simulink model "ASM_Traffic_V2X_Complete_Model_2"  (R2019a)
settings: Solver=ode1  StartTime=SIM.tstart.v  StopTime=Inf  FixedStep=SIM.StepSize.v  RelTol=1e-3
PostLoadFcn:
  | if any(exist('dsrtsu_mdlpostloadfcn', 'file') ~= 0), dsrtsu_mdlpostloadfcn('Execute', bdroot); end
  | try, asm_mdl_postloadfcn(bdroot, 'UpdateModel', 2200); catch, disp(lasterr); end,
undefined symbols (not defined in the file): _SensorPnts_1, _SensorPnts_13, _SensorPnts_17, _SensorPnts_21, _SensorPnts_25, _SensorPnts_29, _SensorPnts_33, _SensorPnts_37, _SensorPnts_41, _SensorPnts_45, _SensorPnts_49, _SensorPnts_5, _SensorPnts_53, _SensorPnts_57, _SensorPnts_9, _to_, CPT, G5A, ITS, MDL, rad, s_to_rpm, SIM
libraries: simulink x169, ASM_VehicleDynamics_lib x126, ASM_Traffic_lib x83, ASM_Utils_lib x49, mdbs x45, ASM_Environment_lib x17, dspindex x12, dsaV2xLibraryAux x10, dsmpblib x6, dsaV2xAsn1Library x4, dsaV2xLibrary x4, ASM_BrakeHydraulics_lib x4
(part 20 of 36)

== system ASM_Traffic_V2X_Complete_Model_2/MDL/Environment/Traffic/Sensors/Custom_Sensor ==
  Fellows_Signals : Inport
  VehicleDynamics_Signals : Inport  Port=2
  Objects_Signals : Inport  Port=3
  Road_Signals : Inport  Port=4
  ASMSignalBus_Mapping : Subsystem
  ASMSignalCollector : Subsystem
  Bus Creator4 : BusCreator  Inputs=1
  Bus Selector : BusSelector  OutputSignals=TrafficObject_Type_Fellows[],TrafficObject_Type_Data[]
  Bus Selector2 : BusSelector  OutputSignals=TrafficObject_Data[]
  Bus Selector3 : BusSelector  OutputSignals=VehicleMovement.Positions.Pos_Vehicle_CoorSys_E[x;y;z][m].Pos_Vehicle_CoorSys_E[x;y;z][m],VehicleMovement.Positions.Angle_Vehicle_CoorSys_E[x;y;z][deg].Angle_Vehicle_CoorSys_E[x;y;z][deg]
  Bus Selector4 : BusSelector  OutputSignals=Pos_Fellows_MainPnt_CoorSys_E[x;y;z][m],Angle_Fellows[x;y;z][deg],Flag_FellowUsed[0|1]
  CUSTOM_SENSOR_GEOMETRY_PARAMETERS : ASM_Traffic_lib/Sensors/Custom_Sensor/CUSTOM_SENSOR_GEOMETRY_PARAMETERS  Tag=ASM_SUBCOMPONENT  Sensor_Enable=MDL.Traffic.Sensors.CustomSensor_Geometry.Sw_Sensor_Enable  Pos_Sensor=MDL.Traffic.Sensors.CustomSensor_Geometry.Const_Pos_Sensor_Apex_CoorSys_V  Angle_Orientation_Sensor=MDL.Traffic.Sensors.CustomSensor_Geometry.Const_Angle_Orientation_Sensor_CoorSys_V  Length_ScopeZone=MDL.Traffic.Sensors.CustomSensor_Geometry.Const_Length_ScopeZone  Angle_ScopeZone_Horizontal=MDL.Traffic.Sensors.CustomSensor_Geometry.Const_Angle_ScopeZone_Horizontal  Angle_ScopeZone_Vertical=MDL.Traffic.Sensors.CustomSensor_Geometry.Const_Angle_ScopeZone_Vertical  ASMProperties=struct('Name','CUSTOM_SENSOR_GEOMETRY_PARAMETERS','Version','2.0','Library','ASM_Traffic_lib')  ASMInstanceName=custom_sensor_geometry_parameters  ASMInstanceID=1
  CUSTOM_SENSOR_OUTPUT : ASM_Traffic_lib/Sensors/Custom_Sensor/CUSTOM_SENSOR_OUTPUT  Tag=ASM_SUBCOMPONENT  ASMProperties=struct('Name','CUSTOM_SENSOR_OUTPUT','Version','4.0','Library','ASM_Traffic_lib')  ASMInstanceName=custom_sensor_output  ASMInstanceID=1
  CUSTOM_SENSOR_SCOPEZONE_CALCULATION : ASM_Traffic_lib/Sensors/Custom_Sensor/CUSTOM_SENSOR_SCOPEZONE_CALCULATION  Tag=ASM_SUBCOMPONENT  ASMProperties=struct('Name','CUSTOM_SENSOR_SCOPEZONE_CALCULATION','Version','4.0','Library','ASM_Traffic_lib')  ASMInstanceName=custom_sensor_scopezone_calculation  ASMInstanceID=1
  Enable_Custom_Sensor : Subsystem
  SensorOutput_Mapping : Subsystem
  TrafficObject_Type : Subsystem
  Vector Concatenate : Concatenate  NumInputs=5
  Sensor_Signals : Outport
  tag scope: ASMBUS_Environment_Traffic_Sensors_Custom_Sensor_1=global, ASMBUS_Environment_Traffic_Sensors_Custom_Sensor_1_Parameters=global
  wires:
  Enable_Custom_Sensor/1(Enable_Out[0Off|1On]) -> CUSTOM_SENSOR_SCOPEZONE_CALCULATION/1
  CUSTOM_SENSOR_GEOMETRY_PARAMETERS/1 -> [ASMBUS_Environment_Traffic_Sensors_Custom_Sensor_1_Parameters]
  TrafficObject_Type/1(Out1) -> CUSTOM_SENSOR_OUTPUT/1
  ASMSignalBus_Mapping/1(ASMSignalBus) -> [ASMBUS_Environment_Traffic_Sensors_Custom_Sensor_1]
  Bus Creator4/1 -> Sensor_Signals/1
  SensorOutput_Mapping/1(Sensor_Signals) -> Bus Creator4/1  "Sensor_Front_1"
  CUSTOM_SENSOR_OUTPUT/2 -> SensorOutput_Mapping/2(ObjectData)
  CUSTOM_SENSOR_SCOPEZONE_CALCULATION/1 -> ASMSignalBus_Mapping/1(ScopezoneData)
  Bus Selector4/1 -> CUSTOM_SENSOR_SCOPEZONE_CALCULATION/5  "<Pos_Fellows_MainPnt_CoorSys_E[x;y;z][m]>"
  CUSTOM_SENSOR_GEOMETRY_PARAMETERS/2 -> Enable_Custom_Sensor/1(Enable_In[0Off|1On])
  CUSTOM_SENSOR_GEOMETRY_PARAMETERS/7 -> Vector Concatenate/5
  CUSTOM_SENSOR_GEOMETRY_PARAMETERS/6 -> Vector Concatenate/4
  CUSTOM_SENSOR_GEOMETRY_PARAMETERS/5 -> Vector Concatenate/3
  CUSTOM_SENSOR_GEOMETRY_PARAMETERS/4 -> Vector Concatenate/2
  CUSTOM_SENSOR_GEOMETRY_PARAMETERS/3 -> Vector Concatenate/1
  Bus Selector4/3 -> CUSTOM_SENSOR_SCOPEZONE_CALCULATION/7  "<Flag_FellowUsed[0|1]>"
  Bus Selector4/2 -> CUSTOM_SENSOR_SCOPEZONE_CALCULATION/6  "<Angle_Fellows[x;y;z][deg]>"
  Bus Selector3/2 -> CUSTOM_SENSOR_SCOPEZONE_CALCULATION/4  "<Angle_Vehicle_CoorSys_E[x;y;z][deg]>"
  Bus Selector3/1 -> CUSTOM_SENSOR_SCOPEZONE_CALCULATION/3  "<Pos_Vehicle_CoorSys_E[x;y;z][m]>"
  Bus Selector2/1 -> CUSTOM_SENSOR_SCOPEZONE_CALCULATION/10  "<TrafficObject_Data[]>"
  Vector Concatenate/1 -> CUSTOM_SENSOR_SCOPEZONE_CALCULATION/2
  Bus Selector/1 -> CUSTOM_SENSOR_SCOPEZONE_CALCULATION/8  "<TrafficObject_Type_Fellows[]>"
  CUSTOM_SENSOR_SCOPEZONE_CALCULATION/2 -> TrafficObject_Type/1(In1), SensorOutput_Mapping/1(ScopezoneData)
  CUSTOM_SENSOR_OUTPUT/1 -> ASMSignalBus_Mapping/2(ObjectData)
  Bus Selector/2 -> CUSTOM_SENSOR_OUTPUT/2, CUSTOM_SENSOR_SCOPEZONE_CALCULATION/9  "<TrafficObject_Type_Data[]>"
  Fellows_Signals/1 -> Bus Selector4/1
  VehicleDynamics_Signals/1 -> Bus Selector3/1
  Objects_Signals/1 -> Bus Selector/1
  Road_Signals/1 -> Bus Selector2/1

== system ASM_Traffic_V2X_Complete_Model_2/MDL/Environment/Traffic/Sensors/Line_Sensor ==
  Enable[0Off|1On] : Inport
  VehicleDynamics_Signals : Inport  Port=2
  Road_Signals : Inport  Port=3
  Maneuver_Signals : Inport  Port=4
  ASMSignalCollector : Subsystem
  Bus Selector1 : BusSelector  OutputSignals=VehicleMovement.Positions.Pos_Vehicle_CoorSys_E[x;y;z][m].Pos_x_Vehicle_CoorSys_E[m],VehicleMovement.Positions.Pos_Vehicle_CoorSys_E[x;y;z][m].Pos_y_Vehicle_CoorSys_E[m],VehicleMovement.Positions.Angle_Vehicle_CoorSys_E[x;y;z][deg].Angle_Yaw_Vehicle_CoorSys_E[deg]
  Bus Selector5 : BusSelector  OutputSignals=MdlControl.Reset_VehicleStates[0|1],Info.ManeuverState[],InitialVehStates.Route_Id_Init[],InitialVehStates.Route_Direction_Init[]
  Bus Selector6 : BusSelector  OutputSignals=Road_ASMVeh.s_Veh_Road[m],Road_Info.d_Veh_Ref_Line[m]
  Enable_Line_Sensor : Subsystem
  LINE_SENSOR : ASM_Traffic_lib/Sensors/Line_Sensor/LINE_SENSOR  Tag=ASM_SUBCOMPONENT  Const_Length_Sensor_Range=MDL.Traffic.Sensors.LineSensor.Const_Length_Sensor_Range  Const_Num_Lines_Per_Side_Max=MDL.Traffic.Sensors.LineSensor.Const_Num_Lines_Per_Side_Max  Const_Dist_Road_Sample_Pnts=MDL.Traffic.Sensors.LineSensor.Const_Dist_Road_Sample_Pnts  Const_Road_Lane_Output_Dimension=MDL.Traffic.Sensors.LineSensor.Const_Road_Lane_Output_Dimension  Const_Road_Shape_Line_Output_Dimension=MDL.Traffic.Sensors.LineSensor.Const_Road_Shape_Line_Output_Dimension  Const_Road_Shape_ContObj_Output_Dimension=MDL.Traffic.Sensors.LineSensor.Const_Road_Shape_ContObj_Output_Dimension  Const_Junction_Border_Output_Dimension=MDL.Traffic.Sensors.LineSensor.Const_Junction_Border_Output_Dimension  Const_Junction_Shape_Line_Output_Dimension=MDL.Traffic.Sensors.LineSensor.Const_Junction_Shape_Line_Output_Dimension  Const_Junction_Shape_ContObj_Output_Dimension=MDL.Traffic.Sensors.LineSensor.Const_Junction_Shape_ContObj_Output_Dimension  Sw_Sensor_Enable=MDL.Traffic.Sensors.LineSensor.Sw_Sensor_Enable  ASMProperties=struct('Name','LINE_SENSOR','Version','5.0','Library','ASM_Traffic_lib')  ASMInstanceName=line_sensor  ASMInstanceID=1
  Sensor_Signals : Outport
  tag scope: ASMBUS_Traf_Sensors_Line_Sensor_1=global
  wires:
  Enable_Line_Sensor/1(Enable_Out[0Off|1On]) -> LINE_SENSOR/1
  Bus Selector6/2 -> LINE_SENSOR/8  "<d_Veh_Ref_Line[m]>"
  Bus Selector1/3 -> LINE_SENSOR/11  "<Angle_Yaw_Vehicle_CoorSys_E[deg]>"
  Bus Selector1/2 -> LINE_SENSOR/10  "<Pos_y_Vehicle_CoorSys_E[m]>"
  Bus Selector1/1 -> LINE_SENSOR/9  "<Pos_x_Vehicle_CoorSys_E[m]>"
  VehicleDynamics_Signals/1 -> Bus Selector1/1
  Bus Selector6/1 -> LINE_SENSOR/7  "<s_Veh_Road[m]>"
  Road_Signals/1 -> Bus Selector6/1
  Bus Selector5/4 -> LINE_SENSOR/6  "<Route_Direction_Init[]>"
  Bus Selector5/3 -> LINE_SENSOR/5  "<Route_Id_Init[]>"
  Bus Selector5/2 -> LINE_SENSOR/4  "<ManeuverState[]>"
  Bus Selector5/1 -> LINE_SENSOR/3  "<Reset_VehicleStates[0|1]>"
  Maneuver_Signals/1 -> Bus Selector5/1
  Enable[0Off|1On]/1 -> Enable_Line_Sensor/1(Enable_In[0Off|1On])
  [ASM_Environment_LineSensorData] -> LINE_SENSOR/2
  LINE_SENSOR/2 -> Sensor_Signals/1
  LINE_SENSOR/1 -> [ASMBUS_Traf_Sensors_Line_Sensor_1]

== system ASM_Traffic_V2X_Complete_Model_2/MDL/Environment/Traffic/Sensors/Object_Sensor_2D ==
  Enable[0Off|1On] : Inport
  Fellows_Signals : Inport  Port=2
  VehicleDynamics_Signals : Inport  Port=3
  Objects_Signals : Inport  Port=4
  Road_Signals : Inport  Port=5
  ASMSignalCollector : Subsystem
  Enable_Object_Sensor_2D : Subsystem
  ScheduleAndCalculateSensor : Subsystem
  SensorMapping : Subsystem
  SensorParameters : Subsystem
  Sensor_Signals : Outport
  wires:
  Enable[0Off|1On]/1 -> Enable_Object_Sensor_2D/1(Enable_In[0Off|1On])
  Enable_Object_Sensor_2D/1(Enable_Out[0Off|1On]) -> ScheduleAndCalculateSensor/2(Enable[0Off|1On]), SensorMapping/1(Enable[0Off|1On])
  SensorMapping/1(Sensor_Signals) -> Sensor_Signals/1
  VehicleDynamics_Signals/1 -> ScheduleAndCalculateSensor/4(VehicleDynamics_Signals)
  SensorParameters/1(Sensor_Data[]) -> ScheduleAndCalculateSensor/1(Sensor_Data[])
  Fellows_Signals/1 -> ScheduleAndCalculateSensor/3(Fellows_Signals)
  Objects_Signals/1 -> ScheduleAndCalculateSensor/5(Objects_Signals)
  Road_Signals/1 -> ScheduleAndCalculateSensor/6(Road_Signals)
  ScheduleAndCalculateSensor/1(SensorMapping_Data[]) -> SensorMapping/2(SensorMapping_Data[])
  ScheduleAndCalculateSensor/2(SensorSignals) -> SensorMapping/3(SensorSignals)

== system ASM_Traffic_V2X_Complete_Model_2/MDL/Environment/Traffic/Sensors/Object_Sensor_3D ==
  Enable[0Off|1On] : Inport
  Fellows_Signals : Inport  Port=2
  VehicleDynamics_Signals : Inport  Port=3
  Objects_Signals : Inport  Port=4
  Road_Signals : Inport  Port=5
  ASMSignalCollector : Subsystem
  CustomPoints : Subsystem
  Enable_Object_Sensor_3D : Subsystem
  RadarEffects : Subsystem
  ScheduleAndCalculateSensor : Subsystem
  SensorMapping : Subsystem
  SensorParameters : Subsystem
  Sensor_Signals : Outport
  wires:
  ScheduleAndCalculateSensor/5(Pos_Vehicle_CoorSys_E_Sampled[x,y;z][m]) -> RadarEffects/5(Pos_Vehicle_CoorSys_E[x;y;z][m])
  ScheduleAndCalculateSensor/4(Angle_Vehicle_CoorSys_E_Sampled[x,y;z][deg]) -> RadarEffects/4(Angle_Vehicle_CoorSys_E[x;y;z][deg])
  ScheduleAndCalculateSensor/3(SensorData[]) -> RadarEffects/3(SensorData[]), CustomPoints/3(SensorData[])
  Enable[0Off|1On]/1 -> Enable_Object_Sensor_3D/1(Enable_In[0Off|1On])
  Enable_Object_Sensor_3D/1(Enable_Out[0Off|1On]) -> ScheduleAndCalculateSensor/2(Enable[0Off|1On]), SensorMapping/1(Enable[0Off|1On]), RadarEffects/1(Enable[0Off|1On]), CustomPoints/1(Enable[0Off|1On])
  SensorMapping/1(Sensor_Signals) -> Sensor_Signals/1
  VehicleDynamics_Signals/1 -> ScheduleAndCalculateSensor/4(VehicleDynamics_Signals)
  SensorParameters/1(Sensor_Data[]) -> ScheduleAndCalculateSensor/1(Sensor_Data[])
  Fellows_Signals/1 -> ScheduleAndCalculateSensor/3(Fellows_Signals)
  Objects_Signals/1 -> ScheduleAndCalculateSensor/5(Objects_Signals)
  Road_Signals/1 -> ScheduleAndCalculateSensor/6(Road_Signals)
  ScheduleAndCalculateSensor/1(SensorMapping_Data[]) -> SensorMapping/2(SensorMapping_Data[]), RadarEffects/2(SensorMapping_Data[]), CustomPoints/2(SensorMapping_Data[])
  ScheduleAndCalculateSensor/2(SensorSignals) -> SensorMapping/3(SensorSignals)

== system ASM_Traffic_V2X_Complete_Model_2/MDL/Environment/Traffic/Sensors/Sensors_Common_Signals ==
  Maneuver_Signals[] : Inport
  Brake : RelationalOperator  Operator===  OutDataTypeStr=boolean  RndMeth=Nearest
  Bus Selector7 : BusSelector  OutputSignals=Info.ManeuverState[]  OutputAsBus=on
  Constant : Constant  Value=3
  Constant1 : Constant  Value=4
  Data Type Conversion : DataTypeConversion  OutDataTypeStr=double
  Delay : Subsystem
  Logical Operator : Logic  Operator=OR  AllPortsSameDT=off  OutDataTypeStr=boolean
  Run : RelationalOperator  Operator===  OutDataTypeStr=boolean  RndMeth=Nearest
  SignalCollector : Subsystem
  ASMSignalBus : Outport
  Enable_Sensor_Scheduling[0Off|1On] : Outport  Port=2
  wires:
  Data Type Conversion/1 -> Delay/1(Enable_Sensor_Scheduling_In[0Off|1On])
  Delay/1(Enable_Sensor_Scheduling_Out[0Off|1On]) -> SignalCollector/1(Enable_SensorScheduling[0Off|1On]), Enable_Sensor_Scheduling[0Off|1On]/1
  SignalCollector/1(ASMSignalBus) -> ASMSignalBus/1
  Logical Operator/1 -> Data Type Conversion/1
  Brake/1 -> Logical Operator/2
  Bus Selector7/1 -> Brake/1, Run/1
  Constant1/1 -> Brake/2
  Run/1 -> Logical Operator/1
  Constant/1 -> Run/2
  Maneuver_Signals[]/1 -> Bus Selector7/1

== system ASM_Traffic_V2X_Complete_Model_2/MDL/Environment/Traffic/Sensors/Traffic_Sign_Sensor ==
  VehicleDynamics_Signals : Inport
  Objects_Signals : Inport  Port=2
  Road_Signals : Inport  Port=3
  ASMSignalCollector : Subsystem
  Bus Selector1 : BusSelector  OutputSignals=VehicleMovement.Positions.Pos_Vehicle_CoorSys_E[x;y;z][m].Pos_Vehicle_CoorSys_E[x;y;z][m],VehicleMovement.Positions.Angle_Vehicle_CoorSys_E[x;y;z][deg].Angle_Vehicle_CoorSys_E[x;y;z][deg]
  Bus Selector2 : BusSelector  OutputSignals=TrafficObject_Type_Data[]
  Bus Selector3 : BusSelector  OutputSignals=TrafficObject_Data[]
  Enable_Traffic_Sign_Sensor : Subsystem
  Mux : Mux  Inputs=6
  Objects_DataStreams : Subsystem
  TRAFFIC_SIGN_SENSOR_DYNAMIC_CALCULATION : ASM_Traffic_lib/Sensors/Traffic_Sign_Sensor/TRAFFIC_SIGN_SENSOR_DYNAMIC_CALCULATION  Tag=ASM_SUBCOMPONENT  Const_Sensor_Output_Dimension=MDL.Traffic.Sensors.TrafficSignSensorDyn_Calculation.Const_Sensor_Output_Dimension  ASMProperties=struct('Name','TRAFFIC_SIGN_SENSOR_DYNAMIC_CALCULATION','Version','1.0','Library','ASM_Traffic_lib')  ASMInstanceName=traffic_sign_sensor_dynamic_calculation  ASMInstanceID=1
  TRAFFIC_SIGN_SENSOR_GEOMETRY_PARAMETERS : ASM_Traffic_lib/Sensors/Traffic_Sign_Sensor/TRAFFIC_SIGN_SENSOR_GEOMETRY_PARAMETERS  Tag=ASM_SUBCOMPONENT  Sensor_Enable=MDL.Traffic.Sensors.TrafficSignSensor_Geometry.Sw_Sensor_Enable  Pos_Sensor=MDL.Traffic.Sensors.TrafficSignSensor_Geometry.Const_Pos_Sensor_Apex_CoorSys_V  Angle_Orientation_Sensor=MDL.Traffic.Sensors.TrafficSignSensor_Geometry.Const_Angle_Orientation_Sensor_CoorSys_V  Length_ScopeZone=MDL.Traffic.Sensors.TrafficSignSensor_Geometry.Const_Length_ScopeZone  Angle_ScopeZone_Horizontal=MDL.Traffic.Sensors.TrafficSignSensor_Geometry.Const_Angle_ScopeZone_Horizontal  Angle_ScopeZone_Vertical=MDL.Traffic.Sensors.TrafficSignSensor_Geometry.Const_Angle_ScopeZone_Vertical  Angle_Sign_Orientation_Max=MDL.Traffic.Sensors.TrafficSignSensor_Geometry.Const_Angle_Sign_Orientation_Max  ASMProperties=struct('Name','TRAFFIC_SIGN_SENSOR_GEOMETRY_PARAMETERS','Version','2.0','Library','ASM_Traffic_lib')  ASMInstanceName=traffic_sign_sensor_geometry_parameters  ASMInstanceID=1
  Sensor_Signals : Outport
  tag scope: ASMBUS_Traf_Sensors_Traffic_Sign_Sensor_dyn_1_Parameters=global, ASMBUS_Traf_Sensors_dyn_Traffic_Sign_Sensor_1=global
  wires:
  Objects_DataStreams/1(TrafficObjects_States[]) -> TRAFFIC_SIGN_SENSOR_DYNAMIC_CALCULATION/7
  Bus Selector3/1 -> TRAFFIC_SIGN_SENSOR_DYNAMIC_CALCULATION/6  "<TrafficObject_Data[]>"
  Bus Selector2/1 -> TRAFFIC_SIGN_SENSOR_DYNAMIC_CALCULATION/5  "<TrafficObject_Type_Data[]>"
  Bus Selector1/2 -> TRAFFIC_SIGN_SENSOR_DYNAMIC_CALCULATION/4  "<Angle_Vehicle_CoorSys_E[x;y;z][deg]>"
  Bus Selector1/1 -> TRAFFIC_SIGN_SENSOR_DYNAMIC_CALCULATION/3  "<Pos_Vehicle_CoorSys_E[x;y;z][m]>"
  TRAFFIC_SIGN_SENSOR_DYNAMIC_CALCULATION/2 -> Sensor_Signals/1
  TRAFFIC_SIGN_SENSOR_DYNAMIC_CALCULATION/1 -> [ASMBUS_Traf_Sensors_dyn_Traffic_Sign_Sensor_1]
  Enable_Traffic_Sign_Sensor/1(Enable_Out[0Off|1On]) -> TRAFFIC_SIGN_SENSOR_DYNAMIC_CALCULATION/1
  TRAFFIC_SIGN_SENSOR_GEOMETRY_PARAMETERS/1 -> [ASMBUS_Traf_Sensors_Traffic_Sign_Sensor_dyn_1_Parameters]
  TRAFFIC_SIGN_SENSOR_GEOMETRY_PARAMETERS/2 -> Enable_Traffic_Sign_Sensor/1(Enable_In[0Off|1On])
  Mux/1 -> TRAFFIC_SIGN_SENSOR_DYNAMIC_CALCULATION/2
  TRAFFIC_SIGN_SENSOR_GEOMETRY_PARAMETERS/8 -> Mux/6
  TRAFFIC_SIGN_SENSOR_GEOMETRY_PARAMETERS/7 -> Mux/5
  TRAFFIC_SIGN_SENSOR_GEOMETRY_PARAMETERS/6 -> Mux/4
  TRAFFIC_SIGN_SENSOR_GEOMETRY_PARAMETERS/5 -> Mux/3
  TRAFFIC_SIGN_SENSOR_GEOMETRY_PARAMETERS/4 -> Mux/2
  TRAFFIC_SIGN_SENSOR_GEOMETRY_PARAMETERS/3 -> Mux/1
  Road_Signals/1 -> Bus Selector3/1
  Objects_Signals/1 -> Bus Selector2/1
  VehicleDynamics_Signals/1 -> Bus Selector1/1

== system ASM_Traffic_V2X_Complete_Model_2/MDL/SoftECU/Map_Inputs/Maneuver/S_R_FlipFlop ==
  S : Inport
  R : Inport  Port=2
  Demux : Demux  Outputs=2
  Logic : CombinatorialLogic  TruthTable=[0 1;1 0;0 1;0 1;1 0;1 0;0 0;0 0]
  Memory : Memory  InitialCondition=initial_condition  InheritSampleTime=on
  Mux : Mux  Inputs=3
  Q : Outport  InitialOutput=0
  !Q : Outport  Port=2  InitialOutput=1
  wires:
  Demux/2 -> !Q/1
  Demux/1 -> Memory/1, Q/1
  S/1 -> Mux/1
  R/1 -> Mux/2
  Memory/1 -> Mux/3
  Mux/1 -> Logic/1
  Logic/1 -> Demux/1

== system ASM_Traffic_V2X_Complete_Model_2/MDL/SoftECU/Map_Inputs/Maneuver/pos_edge_detection ==
  In1 : Inport
  Memory : Memory
  Relational Operator : RelationalOperator  Operator=>  OutDataTypeStr=boolean  RndMeth=Nearest
  Out1 : Outport
  wires:
  Memory/1 -> Relational Operator/2
  Relational Operator/1 -> Out1/1
  In1/1 -> Memory/1, Relational Operator/1

== system ASM_Traffic_V2X_Complete_Model_2/MDL/SoftECU/Map_Inputs/Maneuver/pos_edge_detection1 ==
  In1 : Inport
  Memory : Memory
  Relational Operator : RelationalOperator  Operator=>  OutDataTypeStr=boolean  RndMeth=Nearest
  Out1 : Outport
  wires:
  In1/1 -> Relational Operator/1, Memory/1
  Relational Operator/1 -> Out1/1
  Memory/1 -> Relational Operator/2

== system ASM_Traffic_V2X_Complete_Model_2/MDL/SoftECU/Map_Inputs/Maneuver/pos_edge_detection2 ==
  In1 : Inport
  Memory : Memory
  Relational Operator : RelationalOperator  Operator=>  OutDataTypeStr=boolean  RndMeth=Nearest
  Out1 : Outport
  wires:
  Memory/1 -> Relational Operator/2
  Relational Operator/1 -> Out1/1
  In1/1 -> Memory/1, Relational Operator/1

== system ASM_Traffic_V2X_Complete_Model_2/MDL/SoftECU/Map_Inputs/Maneuver/pos_edge_detection3 ==
  In1 : Inport
  Memory : Memory
  Relational Operator : RelationalOperator  Operator=>  OutDataTypeStr=boolean  RndMeth=Nearest
  Out1 : Outport
  wires:
  In1/1 -> Relational Operator/1, Memory/1
  Relational Operator/1 -> Out1/1
  Memory/1 -> Relational Operator/2

== system ASM_Traffic_V2X_Complete_Model_2/MDL/SoftECU/Soft_ECU_ACC/Map_Inputs/Maneuver ==
  note: Initial value is set
      | to AEBOff (3)
  ECU_Commands[] : Inport
  Reset[0|1] : Inport  Port=2
  ACC_BrakeMode_Default : Constant  Value=3
  Add : Sum  Inputs=+++
  Fcn1 : Fcn  Expr=u(1)==1020
  Fcn10 : Fcn  Expr=u(1)==1031
  Fcn2 : Fcn  Expr=u(1)==1030
  Fcn3 : Fcn  Expr=u(1)==1022
  Fcn4 : Fcn  Expr=u(1)==1021
  Fcn5 : Fcn  Expr=u(1)==1013
  Fcn6 : Fcn  Expr=u(1)==1011
  Fcn7 : Fcn  Expr=u(1)==1010
  Fcn8 : Fcn  Expr=u(1)==1012
  Fcn9 : Fcn  Expr=u(1)==1032
  Gain : Gain
  Gain1 : Gain  Gain=2
  Gain2 : Gain  Gain=3
  Logical Operator : Logic  Operator=OR  Inputs=4  AllPortsSameDT=off  OutDataTypeStr=boolean
  Memory : Memory  InitialCondition=3
  Switch : Switch  Threshold=0.5
  Switch1 : Switch  Threshold=0.5
  pos_edge_detection : Subsystem
  pos_edge_detection1 : Subsystem
  pos_edge_detection2 : Subsystem
  pos_edge_detection3 : Subsystem
  Sw_ACC_On[0Off|1On] : Outport
  Sw_ACC_Off[0Off|1On] : Outport  Port=2
  Sw_ACC_Cancel[0Off|1On] : Outport  Port=3
  Sw_ACC_Resume[0Off|1On] : Outport  Port=4
  Sw_ACC_Speed_Set[0Off|1On] : Outport  Port=5
  Sw_ACC_Speed_Increase[0Off|1On] : Outport  Port=6
  Sw_ACC_Speed_Decrease[0Off|1On] : Outport  Port=7
  Sw_ACC_BrakeMode[1Comfort|2AEBOnly|3AEBOff] : Outport  Port=8
  wires:
  Fcn6/1 -> Sw_ACC_Off[0Off|1On]/1
  Fcn7/1 -> Sw_ACC_On[0Off|1On]/1
  Fcn3/1 -> Sw_ACC_Speed_Decrease[0Off|1On]/1
  Fcn4/1 -> Sw_ACC_Speed_Increase[0Off|1On]/1
  Fcn5/1 -> Sw_ACC_Resume[0Off|1On]/1
  Fcn8/1 -> Sw_ACC_Cancel[0Off|1On]/1
  Fcn1/1 -> Sw_ACC_Speed_Set[0Off|1On]/1
  ECU_Commands[]/1 -> Fcn7/1, Fcn6/1, Fcn8/1, Fcn5/1, Fcn1/1, Fcn4/1, Fcn9/1, Fcn10/1, Fcn2/1, Fcn3/1
  Fcn9/1 -> pos_edge_detection/1(In1), Gain2/1
  Fcn10/1 -> pos_edge_detection1/1(In1), Gain1/1
  Fcn2/1 -> pos_edge_detection2/1(In1), Gain/1
  pos_edge_detection/1(Out1) -> Logical Operator/1
  pos_edge_detection1/1(Out1) -> Logical Operator/2
  pos_edge_detection2/1(Out1) -> Logical Operator/3
  Gain2/1 -> Add/3
  Gain1/1 -> Add/2
  Gain/1 -> Add/1
  Logical Operator/1 -> Switch/2
  Switch/1 -> Sw_ACC_BrakeMode[1Comfort|2AEBOnly|3AEBOff]/1, Memory/1
  Memory/1 -> Switch/3
  pos_edge_detection3/1(Out1) -> Switch1/2, Logical Operator/4
  Add/1 -> Switch1/3
  Reset[0|1]/1 -> pos_edge_detection3/1(In1)
  Switch1/1 -> Switch/1
  ACC_BrakeMode_Default/1 -> Switch1/1

== system ASM_Traffic_V2X_Complete_Model_2/MDL/VehicleDynamics/Brake/BRAKE_HYDRAULICS/ASMSignalCollector ==
  BusCreator : BusCreator  Inputs=2
  Const_BrakeHydraulicsModel[] : Constant  Value=2
      settings: AttributesFormatString=2 - Basic
  ASMSignalBus : Outport
  wires:
  [TAG_DISP_BrkHyd_BrakingCircuitBasic] -> BusCreator/1
  Const_BrakeHydraulicsModel[]/1 -> BusCreator/2  "BrakeHydraulicsModel[]"
  BusCreator/1 -> ASMSignalBus/1  "BrakeHydraulics"

== system ASM_Traffic_V2X_Complete_Model_2/MDL/VehicleDynamics/Suspension/SuspensionFront/ASMSignalCollector ==
  BusCreator1 : BusCreator  Inputs=4
  Terminator_1 : Terminator
  Terminator_2 : Terminator
  tag scope: ASMBUS_SuspensionFront=global
  wires:
  [ASMBUS_SuspensionForcesFront] -> BusCreator1/3
  [ASMBUS_SuspensionComplianceFront] -> BusCreator1/2
  [ASMBUS_WheelRelativePositionFront] -> BusCreator1/4
  [ASMBUS_WheelRelativeVelocityFront] -> Terminator_2/1
  [ASMBUS_SuspensionForcesKinematicsFront] -> Terminator_1/1
  BusCreator1/1 -> [ASMBUS_SuspensionFront]  "SuspensionFront"
  [ASMBUS_SuspensionKinematicsFront] -> BusCreator1/1

== system ASM_Traffic_V2X_Complete_Model_2/MDL/VehicleDynamics/Suspension/SuspensionFront/OpenSusKinFrontModel ==

== system ASM_Traffic_V2X_Complete_Model_2/MDL/VehicleDynamics/Suspension/SuspensionRear/ASMSignalCollector ==
  BusCreator1 : BusCreator  Inputs=4
  Terminator_1 : Terminator
  Terminator_2 : Terminator
  tag scope: ASMBUS_SuspensionRear=global
  wires:
  [ASMBUS_SuspensionForcesRear] -> BusCreator1/3
  [ASMBUS_SuspensionRelativePositionRear] -> BusCreator1/4
  [ASMBUS_SuspensionComplianceRear] -> BusCreator1/2
  [ASMBUS_SuspensionForceKinematicsRear] -> Terminator_2/1
  [ASMBUS_SuspensionRelativeVelocitiesRear] -> Terminator_1/1
  [ASMBUS_SuspensionKinematicsRear] -> BusCreator1/1
  BusCreator1/1 -> [ASMBUS_SuspensionRear]  "SuspensionRear"

== system ASM_Traffic_V2X_Complete_Model_2/MDL/VehicleDynamics/Suspension/SuspensionRear/OpenSusKinRearModel ==

== system ASM_Traffic_V2X_Complete_Model_2/MDL/VehicleDynamics/Tire/ASMSignalCollector/ActiveTire_FL ==
  SW_Tire_Model[1TMEasy|2MF] : Inport
  TMEasy : Inport  Port=2
  MagicFormular : Inport  Port=3
  Bus Selector : BusSelector  OutputSignals=Miscellaneous.v_Circumf_Dyn_FL_Wheel[km|h],Slip.Slip_x_FL[],Slip.Slip_y_FL[],Miscellaneous.r_Dyn_FL_Tire[m],Miscellaneous.CorneringStiffness_FL[N],Miscellaneous.Coef_RollingRes_FL[],Torque.Trq_x_FL_CoorSys_CP[Nm],Torque.Trq_y_FL_CoorSys_W[Nm],Torque.Trq_z_FL_CoorSys_CP[Nm],Force.DynamicForce  OutputAsBus=on
  Bus Selector1 : BusSelector  OutputSignals=Miscellaneous.v_Circumf_Dyn_Wheel[km|h],Slip.Slip_x[],Slip.Slip_y[],Miscellaneous.r_Dyn_Tire[m],Miscellaneous.CorneringStiffness[N],Miscellaneous.Coef_RollingRes[],Torque.Trq_x_CoorSys_CP[Nm],Torque.Trq_y_CoorSys_W[Nm],Torque.Trq_z_CoorSys_CP[Nm],Force  OutputAsBus=on
  Bus2Vec : BusToVector
  Bus2Vec1 : BusToVector
  BusCreator : BusCreator  Inputs=12
  Demux : Demux  Outputs=[1 1 1 1 1 1 1 1 1 1 1 1]
  Multiport Switch10 : MultiPortSwitch  Inputs=2  SaturateOnIntegerOverflow=on
  ASMSignalBus : Outport
  wires:
  Demux/1 -> BusCreator/1  "v_Circumf_Dyn_FL_Wheel[km|h]"
  Demux/2 -> BusCreator/2  "Slip_x_FL[]"
  Demux/3 -> BusCreator/3  "Slip_y_FL[]"
  Demux/4 -> BusCreator/4  "r_Dyn_FL_Tire[m]"
  Demux/5 -> BusCreator/5  "CorneringStiffness_FL[N]"
  Demux/6 -> BusCreator/6  "Coef_RollingRes_FL[]"
  Demux/10 -> BusCreator/10  "F_x_Dyn_FL_Tire_CoorSys_CP[N]"
  Demux/11 -> BusCreator/11  "F_y_Dyn_FL_Tire_CoorSys_CP[N]"
  Demux/12 -> BusCreator/12  "F_z_Dyn_FL_Tire_CoorSys_CP[N]"
  Demux/7 -> BusCreator/7  "Trq_x_FL_CoorSys_CP[Nm]"
  Demux/8 -> BusCreator/8  "Trq_y_FL_CoorSys_W[Nm]"
  Demux/9 -> BusCreator/9  "Trq_z_FL_CoorSys_CP[Nm]"
  Bus2Vec1/1 -> Multiport Switch10/3
  Bus2Vec/1 -> Multiport Switch10/2
  Bus Selector1/1 -> Bus2Vec1/1
  Bus Selector/1 -> Bus2Vec/1
  SW_Tire_Model[1TMEasy|2MF]/1 -> Multiport Switch10/1
  Multiport Switch10/1 -> Demux/1
  BusCreator/1 -> ASMSignalBus/1  "ActiveTire"
  MagicFormular/1 -> Bus Selector1/1
  TMEasy/1 -> Bus Selector/1

== system ASM_Traffic_V2X_Complete_Model_2/MDL/VehicleDynamics/Tire/ASMSignalCollector/ActiveTire_FR ==
  SW_Tire_Model[1TMEasy|2MF] : Inport
  TMEasy : Inport  Port=2
  MagicFormular : Inport  Port=3
  Bus Selector : BusSelector  OutputSignals=Miscellaneous.v_Circumf_Dyn_FR_Wheel[km|h],Slip.Slip_x_FR[],Slip.Slip_y_FR[],Miscellaneous.r_Dyn_FR_Tire[m],Miscellaneous.CorneringStiffness_FR[N],Miscellaneous.Coef_RollingRes_FR[],Torque.Trq_x_FR_CoorSys_CP[Nm],Torque.Trq_y_FR_CoorSys_W[Nm],Torque.Trq_z_FR_CoorSys_CP[Nm],Force.DynamicForce  OutputAsBus=on
  Bus Selector1 : BusSelector  OutputSignals=Miscellaneous.v_Circumf_Dyn_Wheel[km|h],Slip.Slip_x[],Slip.Slip_y[],Miscellaneous.r_Dyn_Tire[m],Miscellaneous.CorneringStiffness[N],Miscellaneous.Coef_RollingRes[],Torque.Trq_x_CoorSys_CP[Nm],Torque.Trq_y_CoorSys_W[Nm],Torque.Trq_z_CoorSys_CP[Nm],Force  OutputAsBus=on
  Bus2Vec : BusToVector
  Bus2Vec1 : BusToVector
  BusCreator : BusCreator  Inputs=12
  Demux : Demux  Outputs=[1 1 1 1 1 1 1 1 1 1 1 1]
  Multiport Switch10 : MultiPortSwitch  Inputs=2  SaturateOnIntegerOverflow=on
  ASMSignalBus : Outport
  wires:
  Multiport Switch10/1 -> Demux/1
  Demux/9 -> BusCreator/9  "Trq_z_FR_CoorSys_CP[Nm]"
  Demux/8 -> BusCreator/8  "Trq_y_FR_CoorSys_W[Nm]"
  Demux/7 -> BusCreator/7  "Trq_x_FR_CoorSys_CP[Nm]"
  Demux/12 -> BusCreator/12  "F_z_Dyn_FR_Tire_CoorSys_CP[N]"
  Demux/11 -> BusCreator/11  "F_y_Dyn_FR_Tire_CoorSys_CP[N]"
  Demux/10 -> BusCreator/10  "F_x_Dyn_FR_Tire_CoorSys_CP[N]"
  Demux/6 -> BusCreator/6  "Coef_RollingRes_FR[]"
  Demux/5 -> BusCreator/5  "CorneringStiffness_FR[N]"
  Demux/4 -> BusCreator/4  "r_Dyn_FR_Tire[m]"
  Demux/3 -> BusCreator/3  "Slip_y_FR[]"
  Demux/2 -> BusCreator/2  "Slip_x_FR[]"
  Demux/1 -> BusCreator/1  "v_Circumf_Dyn_FR_Wheel[km|h]"
  Bus2Vec1/1 -> Multiport Switch10/3
  Bus2Vec/1 -> Multiport Switch10/2
  Bus Selector1/1 -> Bus2Vec1/1
  Bus Selector/1 -> Bus2Vec/1
  SW_Tire_Model[1TMEasy|2MF]/1 -> Multiport Switch10/1
  TMEasy/1 -> Bus Selector/1
  MagicFormular/1 -> Bus Selector1/1
  BusCreator/1 -> ASMSignalBus/1  "ActiveTire"

== system ASM_Traffic_V2X_Complete_Model_2/MDL/VehicleDynamics/Tire/ASMSignalCollector/ActiveTire_RL ==
  SW_Tire_Model[1TMEasy|2MF] : Inport
  TMEasy : Inport  Port=2
  MagicFormular : Inport  Port=3
  Bus Selector : BusSelector  OutputSignals=Miscellaneous.v_Circumf_Dyn_RL_Wheel[km|h],Slip.Slip_x_RL[],Slip.Slip_y_RL[],Miscellaneous.r_Dyn_RL_Tire[m],Miscellaneous.CorneringStiffness_RL[N],Miscellaneous.Coef_RollingRes_RL[],Torque.Trq_x_RL_CoorSys_CP[Nm],Torque.Trq_y_RL_CoorSys_W[Nm],Torque.Trq_z_RL_CoorSys_CP[Nm],Force.DynamicForce  OutputAsBus=on
  Bus Selector1 : BusSelector  OutputSignals=Miscellaneous.v_Circumf_Dyn_Wheel[km|h],Slip.Slip_x[],Slip.Slip_y[],Miscellaneous.r_Dyn_Tire[m],Miscellaneous.CorneringStiffness[N],Miscellaneous.Coef_RollingRes[],Torque.Trq_x_CoorSys_CP[Nm],Torque.Trq_y_CoorSys_W[Nm],Torque.Trq_z_CoorSys_CP[Nm],Force  OutputAsBus=on
  Bus2Vec : BusToVector
  Bus2Vec1 : BusToVector
  BusCreator : BusCreator  Inputs=12
  Demux : Demux  Outputs=[1 1 1 1 1 1 1 1 1 1 1 1]
  Multiport Switch10 : MultiPortSwitch  Inputs=2  SaturateOnIntegerOverflow=on
  ASMSignalBus : Outport
  wires:
  Bus2Vec1/1 -> Multiport Switch10/3
  Bus2Vec/1 -> Multiport Switch10/2
  Demux/1 -> BusCreator/1  "v_Circumf_Dyn_RL_Wheel[km|h]"
  Demux/2 -> BusCreator/2  "Slip_x_RL[]"
  Demux/3 -> BusCreator/3  "Slip_y_RL[]"
  Demux/4 -> BusCreator/4  "r_Dyn_RL_Tire[m]"
  Demux/5 -> BusCreator/5  "CorneringStiffness_RL[N]"
  Demux/6 -> BusCreator/6  "Coef_RollingRes_RL[]"
  Demux/10 -> BusCreator/10  "F_x_Dyn_RL_Tire_CoorSys_CP[N]"
  Demux/11 -> BusCreator/11  "F_y_Dyn_RL_Tire_CoorSys_CP[N]"
  Demux/12 -> BusCreator/12  "F_z_Dyn_RL_Tire_CoorSys_CP[N]"
  Demux/7 -> BusCreator/7  "Trq_x_RL_CoorSys_CP[Nm]"
  Demux/8 -> BusCreator/8  "Trq_y_RL_CoorSys_W[Nm]"
  Demux/9 -> BusCreator/9  "Trq_z_RL_CoorSys_CP[Nm]"
  Multiport Switch10/1 -> Demux/1
  Bus Selector1/1 -> Bus2Vec1/1
  Bus Selector/1 -> Bus2Vec/1
  SW_Tire_Model[1TMEasy|2MF]/1 -> Multiport Switch10/1
  BusCreator/1 -> ASMSignalBus/1  "ActiveTire"
  MagicFormular/1 -> Bus Selector1/1
  TMEasy/1 -> Bus Selector/1

== system ASM_Traffic_V2X_Complete_Model_2/MDL/VehicleDynamics/Tire/ASMSignalCollector/ActiveTire_RR ==
  SW_Tire_Model[1TMEasy|2MF] : Inport
  TMEasy : Inport  Port=2
  MagicFormular : Inport  Port=3
  Bus Selector : BusSelector  OutputSignals=Miscellaneous.v_Circumf_Dyn_RR_Wheel[km|h],Slip.Slip_x_RR[],Slip.Slip_y_RR[],Miscellaneous.r_Dyn_RR_Tire[m],Miscellaneous.CorneringStiffness_RR[N],Miscellaneous.Coef_RollingRes_RR[],Torque.Trq_x_RR_CoorSys_CP[Nm],Torque.Trq_y_RR_CoorSys_W[Nm],Torque.Trq_z_RR_CoorSys_CP[Nm],Force.DynamicForce  OutputAsBus=on
  Bus Selector1 : BusSelector  OutputSignals=Miscellaneous.v_Circumf_Dyn_Wheel[km|h],Slip.Slip_x[],Slip.Slip_y[],Miscellaneous.r_Dyn_Tire[m],Miscellaneous.CorneringStiffness[N],Miscellaneous.Coef_RollingRes[],Torque.Trq_x_CoorSys_CP[Nm],Torque.Trq_y_CoorSys_W[Nm],Torque.Trq_z_CoorSys_CP[Nm],Force  OutputAsBus=on
  Bus2Vec : BusToVector
  Bus2Vec1 : BusToVector
  BusCreator1 : BusCreator  Inputs=12
  Demux : Demux  Outputs=[1 1 1 1 1 1 1 1 1 1 1 1]
  Multiport Switch10 : MultiPortSwitch  Inputs=2  SaturateOnIntegerOverflow=on
  ASMSignalBus : Outport
  wires:
  Bus2Vec1/1 -> Multiport Switch10/3
  Bus2Vec/1 -> Multiport Switch10/2
  Multiport Switch10/1 -> Demux/1
  Demux/9 -> BusCreator1/9  "Trq_z_RR_CoorSys_CP[Nm]"
  Demux/8 -> BusCreator1/8  "Trq_y_RR_CoorSys_W[Nm]"
  Demux/7 -> BusCreator1/7  "Trq_x_RR_CoorSys_CP[Nm]"
  Demux/12 -> BusCreator1/12  "F_z_Dyn_RR_Tire_CoorSys_CP[N]"
  Demux/11 -> BusCreator1/11  "F_y_Dyn_RR_Tire_CoorSys_CP[N]"
  Demux/10 -> BusCreator1/10  "F_x_Dyn_RR_Tire_CoorSys_CP[N]"
  Demux/6 -> BusCreator1/6  "Coef_RollingRes_RR[]"
  Demux/5 -> BusCreator1/5  "CorneringStiffness_RR[N]"
  Demux/4 -> BusCreator1/4  "r_Dyn_RR_Tire[m]"
  Demux/3 -> BusCreator1/3  "Slip_y_RR[]"
  Demux/2 -> BusCreator1/2  "Slip_x_RR[]"
  Demux/1 -> BusCreator1/1  "v_Circumf_Dyn_RR_Wheel[km|h]"
  Bus Selector1/1 -> Bus2Vec1/1
  Bus Selector/1 -> Bus2Vec/1
  SW_Tire_Model[1TMEasy|2MF]/1 -> Multiport Switch10/1
  TMEasy/1 -> Bus Selector/1
  MagicFormular/1 -> Bus Selector1/1
  BusCreator1/1 -> ASMSignalBus/1  "ActiveTire"

== system ASM_Traffic_V2X_Complete_Model_2/MDLUserInterface/Drivetrain/MDL_DISP/ActiveTransmission/Inertia_Trm[kgm2] ==
  In1 : Inport
  Out1 : Outport
  wires:
  In1/1 -> Out1/1

== system ASM_Traffic_V2X_Complete_Model_2/MDLUserInterface/Drivetrain/MDL_DISP/ActiveTransmission/Trq_Out_Trm[Nm] ==
  In1 : Inport
  Out1 : Outport
  wires:
  In1/1 -> Out1/1

== system ASM_Traffic_V2X_Complete_Model_2/MDLUserInterface/Drivetrain/MDL_DISP/ActiveTransmission/i_Trm[] ==
  In1 : Inport
  Out1 : Outport
  wires:
  In1/1 -> Out1/1

== system ASM_Traffic_V2X_Complete_Model_2/MDLUserInterface/Drivetrain/MDL_DISP/ActiveTransmission/i_unsync_Trm[] ==
  In1 : Inport
  Out1 : Outport
  wires:
  In1/1 -> Out1/1

== system ASM_Traffic_V2X_Complete_Model_2/MDLUserInterface/Drivetrain/MDL_DISP/ActiveTransmission/omega_In_Trm[rad|s] ==
  In1 : Inport
  Out1 : Outport
  wires:
  In1/1 -> Out1/1

== system ASM_Traffic_V2X_Complete_Model_2/MDLUserInterface/Drivetrain/MDL_DISP/ActiveTransmission/omega_Out_Trm[rad|s] ==
  In1 : Inport
  Out1 : Outport
  wires:
  In1/1 -> Out1/1

== system ASM_Traffic_V2X_Complete_Model_2/MDLUserInterface/Drivetrain/MDL_DISP/AutomaticTransmission/Trq_Fric_Clutch[Nm] ==
  In1 : Inport
  Out1 : Outport
  wires:
  In1/1 -> Out1/1

== system ASM_Traffic_V2X_Complete_Model_2/MDLUserInterface/Drivetrain/MDL_DISP/AutomaticTransmission/Trq_Pump[Nm] ==
  In1 : Inport
  Out1 : Outport
  wires:
  In1/1 -> Out1/1

== system ASM_Traffic_V2X_Complete_Model_2/MDLUserInterface/Drivetrain/MDL_DISP/AutomaticTransmission/Trq_TorsionSpring_Clutch[Nm] ==
  In1 : Inport
  Out1 : Outport
  wires:
  In1/1 -> Out1/1

== system ASM_Traffic_V2X_Complete_Model_2/MDLUserInterface/Drivetrain/MDL_DISP/AutomaticTransmission/Trq_Turbine[Nm] ==
  In1 : Inport
  Out1 : Outport
  wires:
  In1/1 -> Out1/1

== system ASM_Traffic_V2X_Complete_Model_2/MDLUserInterface/Drivetrain/MDL_DISP/AutomaticTransmission/omega_Out_ClutchPlate[rad|s] ==
  In1 : Inport
  Out1 : Outport
  wires:
  In1/1 -> Out1/1

== system ASM_Traffic_V2X_Complete_Model_2/MDLUserInterface/Drivetrain/MDL_DISP/EngineSpeed/Trq_Starter[Nm] ==
  In1 : Inport
  Out1 : Outport
  wires:
  In1/1 -> Out1/1

== system ASM_Traffic_V2X_Complete_Model_2/MDLUserInterface/Drivetrain/MDL_DISP/EngineSpeed/n_Engine[rpm] ==
  In1 : Inport
  Out1 : Outport
  wires:
  In1/1 -> Out1/1

== system ASM_Traffic_V2X_Complete_Model_2/MDLUserInterface/Drivetrain/MDL_DISP/ManualTransmission/Trq_Fric_Clutch[Nm] ==
  In1 : Inport
  Out1 : Outport
  wires:
  In1/1 -> Out1/1

== system ASM_Traffic_V2X_Complete_Model_2/MDLUserInterface/Drivetrain/MDL_DISP/ManualTransmission/Trq_TorsionSpring_Clutch[Nm] ==
  In1 : Inport
  Out1 : Outport
  wires:
  In1/1 -> Out1/1

== system ASM_Traffic_V2X_Complete_Model_2/MDLUserInterface/Drivetrain/MDL_DISP/ManualTransmission/omega_Out_ClutchPlate[rad|s] ==
  In1 : Inport
  Out1 : Outport
  wires:
  In1/1 -> Out1/1

== system ASM_Traffic_V2X_Complete_Model_2/MDLUserInterface/Drivetrain/MDL_DISP/Shafts/Trq_CF_Shaft[Nm] ==
  In1 : Inport
  Out1 : Outport
  wires:
  In1/1 -> Out1/1

== system ASM_Traffic_V2X_Complete_Model_2/MDLUserInterface/Drivetrain/MDL_DISP/Shafts/Trq_CR_Shaft[Nm] ==
  In1 : Inport
  Out1 : Outport
  wires:
  In1/1 -> Out1/1

== system ASM_Traffic_V2X_Complete_Model_2/MDLUserInterface/Drivetrain/MDL_DISP/Shafts/Trq_FL_Shaft[Nm] ==
  In1 : Inport
  Out1 : Outport
  wires:
  In1/1 -> Out1/1

== system ASM_Traffic_V2X_Complete_Model_2/MDLUserInterface/Drivetrain/MDL_DISP/Shafts/Trq_FR_Shaft[Nm] ==
  In1 : Inport
  Out1 : Outport
  wires:
  In1/1 -> Out1/1

== system ASM_Traffic_V2X_Complete_Model_2/MDLUserInterface/Drivetrain/MDL_DISP/Shafts/Trq_RL_Shaft[Nm] ==
  In1 : Inport
  Out1 : Outport
  wires:
  In1/1 -> Out1/1

== system ASM_Traffic_V2X_Complete_Model_2/MDLUserInterface/Drivetrain/MDL_DISP/Shafts/Trq_RR_Shaft[Nm] ==
  In1 : Inport
  Out1 : Outport
  wires:
  In1/1 -> Out1/1

== system ASM_Traffic_V2X_Complete_Model_2/MDLUserInterface/Environment/MDL_DISP/Driver/AbsoluteError ==
  Current : Inport
  Set : Inport  Port=2
  Sum : Sum  Inputs=|+-  SaturateOnIntegerOverflow=on  InputSameDT=on  OutDataTypeStr=Inherit: Same as first input
  AbsoluteError[km|h] : Outport
  wires:
  Sum/1 -> AbsoluteError[km|h]/1
  Set/1 -> Sum/2
  Current/1 -> Sum/1

== system ASM_Traffic_V2X_Complete_Model_2/MDLUserInterface/Environment/MDL_DISP/Driver/Angle_SteeringWheel[deg] ==
  In1 : Inport
  Out1 : Outport
  wires:
  In1/1 -> Out1/1

== system ASM_Traffic_V2X_Complete_Model_2/MDLUserInterface/Environment/MDL_DISP/Driver/Gear[] ==
  In1 : Inport
  Out1 : Outport
  wires:
  In1/1 -> Out1/1

== system ASM_Traffic_V2X_Complete_Model_2/MDLUserInterface/Environment/MDL_DISP/Driver/Pos_AccPedal[%] ==
  In1 : Inport
  Out1 : Outport
  wires:
  In1/1 -> Out1/1

== system ASM_Traffic_V2X_Complete_Model_2/MDLUserInterface/Environment/MDL_DISP/Driver/Pos_BrakePedal[%] ==
  In1 : Inport
  Out1 : Outport
  wires:
  In1/1 -> Out1/1

== system ASM_Traffic_V2X_Complete_Model_2/MDLUserInterface/Environment/MDL_DISP/Driver/Pos_ClutchPedal[%] ==
  In1 : Inport
  Out1 : Outport
  wires:
  In1/1 -> Out1/1

== system ASM_Traffic_V2X_Complete_Model_2/MDLUserInterface/Environment/MDL_DISP/Driver/RelativeError ==
  Current : Inport
  Set : Inport  Port=2
  AvoidNAN : Fcn  Expr=u/(u*u+1.E-20)
  Limit_RelativeError : Saturate  UpperLimit=UpLim  LowerLimit=LowLim
  Product : Product  SaturateOnIntegerOverflow=on  InputSameDT=on  OutDataTypeStr=Inherit: Same as first input
  Sum : Sum  Inputs=|+-  SaturateOnIntegerOverflow=on  InputSameDT=on  OutDataTypeStr=Inherit: Same as first input
  "[0_1]2[%]" : Gain  Gain=100  SaturateOnIntegerOverflow=on  OutDataTypeStr=Inherit: Same as input  ParamDataTypeStr=Inherit: Same as input
  RelativeError[%] : Outport
  wires:
  Limit_RelativeError/1 -> RelativeError[%]/1
  "[0_1]2[%]"/1 -> Limit_RelativeError/1
  Sum/1 -> Product/1
  Set/1 -> Sum/2, AvoidNAN/1
  Product/1 -> "[0_1]2[%]"/1
  Current/1 -> Sum/1
  AvoidNAN/1 -> Product/2

== system ASM_Traffic_V2X_Complete_Model_2/MDLUserInterface/Environment/MDL_DISP/Driver/SelectorLever[-3T|-2P|-1R|0N|1D] ==
  In1 : Inport
  Out1 : Outport
  wires:
  In1/1 -> Out1/1

== system ASM_Traffic_V2X_Complete_Model_2/MDLUserInterface/Environment/MDL_DISP/Driver/a_x_Vehicle_Ref[m|s2] ==
  In1 : Inport
  Out1 : Outport
  wires:
  In1/1 -> Out1/1

== system ASM_Traffic_V2X_Complete_Model_2/MDLUserInterface/Environment/MDL_DISP/Driver/e_Lat[m] ==
  In1 : Inport
  Out1 : Outport
  wires:
  In1/1 -> Out1/1

== system ASM_Traffic_V2X_Complete_Model_2/MDLUserInterface/Environment/MDL_DISP/Driver/v_Vehicle_Ref[km|h] ==
  In1 : Inport
  Out1 : Outport
  wires:
  In1/1 -> Out1/1

== system ASM_Traffic_V2X_Complete_Model_2/MDLUserInterface/Environment/MDL_DISP/Driver/v_x_Vehicle_CoG[km|h] ==
  In1 : Inport
  Out1 : Outport
  wires:
  In1/1 -> Out1/1

== system ASM_Traffic_V2X_Complete_Model_2/MDLUserInterface/Environment/MDL_DISP/Maneuver/CurrentSegment[] ==
  In1 : Inport
  Out1 : Outport
  wires:
  In1/1 -> Out1/1

== system ASM_Traffic_V2X_Complete_Model_2/MDLUserInterface/Environment/MDL_DISP/Maneuver/ManeuverState[] ==
  In1 : Inport
  Out1 : Outport
  wires:
  In1/1 -> Out1/1

== system ASM_Traffic_V2X_Complete_Model_2/MDLUserInterface/Environment/MDL_DISP/Maneuver/ManeuverTime[s] ==
  In1 : Inport
  Out1 : Outport
  wires:
  In1/1 -> Out1/1

== system ASM_Traffic_V2X_Complete_Model_2/MDLUserInterface/Environment/MDL_DISP/Maneuver/Road_Mode[1NoRoad|2Straight|3Circle|4Road] ==
  In1 : Inport
  Out1 : Outport
  wires:
  In1/1 -> Out1/1

== system ASM_Traffic_V2X_Complete_Model_2/MDLUserInterface/Environment/MDL_DISP/Maneuver/s_local[m] ==
  In1 : Inport
  Out1 : Outport
  wires:
  In1/1 -> Out1/1

== system ASM_Traffic_V2X_Complete_Model_2/MDLUserInterface/Environment/MDL_DISP/Maneuver/t_local[s] ==
  In1 : Inport
  Out1 : Outport
  wires:
  In1/1 -> Out1/1

== system ASM_Traffic_V2X_Complete_Model_2/MDLUserInterface/Environment/MDL_DISP/Road/Angle_Yaw_Veh_Road[deg] ==
  In1 : Inport
  Out1 : Outport
  wires:
  In1/1 -> Out1/1

== system ASM_Traffic_V2X_Complete_Model_2/MDLUserInterface/Environment/MDL_DISP/Road/Curv_Veh_Road[1|m] ==
  In1 : Inport
  Out1 : Outport
  wires:
  In1/1 -> Out1/1

== system ASM_Traffic_V2X_Complete_Model_2/MDLUserInterface/Environment/MDL_DISP/Road/Distance_Marker_Left[m] ==
  In1 : Inport
  Out1 : Outport
  wires:
  In1/1 -> Out1/1

== system ASM_Traffic_V2X_Complete_Model_2/MDLUserInterface/Environment/MDL_DISP/Road/Distance_Marker_Right[m] ==
  In1 : Inport
  Out1 : Outport
  wires:
  In1/1 -> Out1/1

== system ASM_Traffic_V2X_Complete_Model_2/MDLUserInterface/Environment/MDL_DISP/Road/Distance_MeasPnt1_Marker_Left[m] ==
  In1 : Inport
  Out1 : Outport
  wires:
  In1/1 -> Out1/1

== system ASM_Traffic_V2X_Complete_Model_2/MDLUserInterface/Environment/MDL_DISP/Road/Distance_MeasPnt1_Marker_Right[m] ==
  In1 : Inport
  Out1 : Outport
  wires:
  In1/1 -> Out1/1

== system ASM_Traffic_V2X_Complete_Model_2/MDLUserInterface/Environment/MDL_DISP/Road/Distance_MeasPnt2_Marker_Left[m] ==
  In1 : Inport
  Out1 : Outport
  wires:
  In1/1 -> Out1/1

== system ASM_Traffic_V2X_Complete_Model_2/MDLUserInterface/Environment/MDL_DISP/Road/Distance_MeasPnt2_Marker_Right[m] ==
  In1 : Inport
  Out1 : Outport
  wires:
  In1/1 -> Out1/1

== system ASM_Traffic_V2X_Complete_Model_2/MDLUserInterface/Environment/MDL_DISP/Road/Fric_Coeff_CP[:][] ==
  In1 : Inport
  Out1 : Outport
  wires:
  In1/1 -> Out1/1

== system ASM_Traffic_V2X_Complete_Model_2/MDLUserInterface/Environment/MDL_DISP/Road/GPS_Latitude_Road[deg] ==
  In1 : Inport
  Out1 : Outport
  wires:
  In1/1 -> Out1/1

== system ASM_Traffic_V2X_Complete_Model_2/MDLUserInterface/Environment/MDL_DISP/Road/GPS_Longitude_Road[deg] ==
  In1 : Inport
  Out1 : Outport
  wires:
  In1/1 -> Out1/1

== system ASM_Traffic_V2X_Complete_Model_2/MDLUserInterface/Environment/MDL_DISP/Road/LaneWidth[m] ==
  In1 : Inport
  Out1 : Outport
  wires:
  In1/1 -> Out1/1

== system ASM_Traffic_V2X_Complete_Model_2/MDLUserInterface/Environment/MDL_DISP/Road/MarkerType_Left[] ==
  In1 : Inport
  Out1 : Outport
  wires:
  In1/1 -> Out1/1

== system ASM_Traffic_V2X_Complete_Model_2/MDLUserInterface/Environment/MDL_DISP/Road/MarkerType_Right[] ==
  In1 : Inport
  Out1 : Outport
  wires:
  In1/1 -> Out1/1

== system ASM_Traffic_V2X_Complete_Model_2/MDLUserInterface/Environment/MDL_DISP/Road/Pos_x_Ref_Veh_Road[m] ==
  In1 : Inport
  Out1 : Outport
  wires:
  In1/1 -> Out1/1

== system ASM_Traffic_V2X_Complete_Model_2/MDLUserInterface/Environment/MDL_DISP/Road/Pos_y_Ref_Veh_Road[m] ==
  In1 : Inport
  Out1 : Outport
  wires:
  In1/1 -> Out1/1

== system ASM_Traffic_V2X_Complete_Model_2/MDLUserInterface/Environment/MDL_DISP/Road/Pos_z_CP[:][m] ==
  In1 : Inport
  Out1 : Outport
  wires:
  In1/1 -> Out1/1

== system ASM_Traffic_V2X_Complete_Model_2/MDLUserInterface/Environment/MDL_DISP/Road/Slope_Veh_Road[%] ==
  In1 : Inport
  Out1 : Outport
  wires:
  In1/1 -> Out1/1

== system ASM_Traffic_V2X_Complete_Model_2/MDLUserInterface/Environment/MDL_DISP/Road/Sw_Tire_Parameter_Set_CP[:][1|2|3|4] ==
  In1 : Inport
  Out1 : Outport
  wires:
  In1/1 -> Out1/1

== system ASM_Traffic_V2X_Complete_Model_2/MDLUserInterface/Environment/MDL_DISP/Road/Velocity_MeasPnt1_Marker_Left[m|s] ==
  In1 : Inport
  Out1 : Outport
  wires:
  In1/1 -> Out1/1

== system ASM_Traffic_V2X_Complete_Model_2/MDLUserInterface/Environment/MDL_DISP/Road/Velocity_MeasPnt1_Marker_Right[m|s] ==
  In1 : Inport
  Out1 : Outport
  wires:
  In1/1 -> Out1/1

== system ASM_Traffic_V2X_Complete_Model_2/MDLUserInterface/Environment/MDL_DISP/Road/Velocity_MeasPnt2_Marker_Left[m|s] ==
  In1 : Inport
  Out1 : Outport
  wires:
  In1/1 -> Out1/1

== system ASM_Traffic_V2X_Complete_Model_2/MDLUserInterface/Environment/MDL_DISP/Road/Velocity_MeasPnt2_Marker_Right[m|s] ==
  In1 : Inport
  Out1 : Outport
  wires:
  In1/1 -> Out1/1

== system ASM_Traffic_V2X_Complete_Model_2/MDLUserInterface/Environment/MDL_DISP/Road/s_Veh_Road[m] ==
  In1 : Inport
  Out1 : Outport
  wires:
  In1/1 -> Out1/1

== system ASM_Traffic_V2X_Complete_Model_2/MDLUserInterface/Environment/MDL_DISP/Traffic/Custom_Sensor ==
  TrafficBus : Inport
  Angle_Hor_Rel[deg] : Subsystem
      mask Display: disp('')
  Angle_Hor_Rel[deg]1 : Subsystem
      mask Display: disp('')
  Angle_Ver_Rel[deg] : Subsystem
      mask Display: disp('')
  Angle_Ver_Rel[deg]1 : Subsystem
      mask Display: disp('')
  Bus Selector1 : BusSelector  OutputSignals=Sensors.Custom_Sensor.Sensor_Front_1
  Bus Selector2 : BusSelector  OutputSignals=Info.CustomSensor_ScopezoneSfcn_State[],Info.CustomSensor_OutputSfcn_State[],Info.CustomSensor_Data_Valid[0|1]
  Bus Selector3 : BusSelector  OutputSignals=SensorOutput.Object1
  Bus Selector4 : BusSelector  OutputSignals=Object_Valid[0|1],Object_ID[],Object_Type[],Distance[m],Angle_Hor_Rel[deg],Angle_Ver_Rel[deg],CustomValues[]
  Bus Selector5 : BusSelector  OutputSignals=SensorOutput.Object1
  Bus Selector6 : BusSelector  OutputSignals=Object_Valid[0|1],Object_ID[],Object_Type[],Distance[m],Angle_Hor_Rel[deg],Angle_Ver_Rel[deg],CustomValues[]
  CustomSensor_Data_Valid[0|1] : Subsystem
      mask Display: disp('')
  CustomSensor_OutputSfcn_State[] : Subsystem
      mask Display: disp('')
  CustomSensor_ScopezoneSfcn_State[] : Subsystem
      mask Display: disp('')
  CustomValues[] : Subsystem
      mask Display: disp('')
  CustomValues[]1 : Subsystem
      mask Display: disp('')
  Custom_Sensor_Info : Scope  NumInputPorts=3
  Custom_Sensor_Measurement_Object_1 : Scope  NumInputPorts=7
  Custom_Sensor_Measurement_Object_2 : Scope  NumInputPorts=7
  Distance[m] : Subsystem
      mask Display: disp('')
  Distance[m]1 : Subsystem
      mask Display: disp('')
  Object_ID[] : Subsystem
      mask Display: disp('')
  Object_ID[]1 : Subsystem
      mask Display: disp('')
  Object_Type[] : Subsystem
      mask Display: disp('')
  Object_Type[]1 : Subsystem
      mask Display: disp('')
  Object_Valid[0|1] : Subsystem
      mask Display: disp('')
  Object_Valid[0|1]1 : Subsystem
      mask Display: disp('')
  wires:
  Angle_Ver_Rel[deg]/1(Out1) -> Custom_Sensor_Measurement_Object_1/6  "Angle_Ver_Rel[deg]"
  Angle_Hor_Rel[deg]/1(Out1) -> Custom_Sensor_Measurement_Object_1/5  "Angle_Hor_Rel[deg]"
  Distance[m]/1(Out1) -> Custom_Sensor_Measurement_Object_1/4  "Distance[m]"
  Object_Valid[0|1]/1(Out1) -> Custom_Sensor_Measurement_Object_1/1  "Object_Valid[0|1]"
  Bus Selector4/6 -> Angle_Ver_Rel[deg]/1(In1)  "<Angle_Ver_Rel[deg]>"
  Bus Selector4/5 -> Angle_Hor_Rel[deg]/1(In1)  "<Angle_Hor_Rel[deg]>"
  Bus Selector4/4 -> Distance[m]/1(In1)  "<Distance[m]>"
  Bus Selector4/3 -> Object_Type[]/1(In1)  "<Object_Type[]>"
  Bus Selector4/2 -> Object_ID[]/1(In1)  "<Object_ID[]>"
  Bus Selector4/1 -> Object_Valid[0|1]/1(In1)  "<Object_Valid[0|1]>"
  CustomSensor_OutputSfcn_State[]/1(Out1) -> Custom_Sensor_Info/2  "CustomSensor_OutputSfcn_State[]"
  CustomSensor_ScopezoneSfcn_State[]/1(Out1) -> Custom_Sensor_Info/1  "CustomSensor_ScopezoneSfcn_State[]"
  Bus Selector2/2 -> CustomSensor_OutputSfcn_State[]/1(In1)  "<CustomSensor_OutputSfcn_State[]>"
  Bus Selector2/1 -> CustomSensor_ScopezoneSfcn_State[]/1(In1)  "<CustomSensor_ScopezoneSfcn_State[]>"
  Bus Selector1/1 -> Bus Selector5/1, Bus Selector3/1, Bus Selector2/1  "<Sensor_Front_1>"
  TrafficBus/1 -> Bus Selector1/1
  Object_ID[]/1(Out1) -> Custom_Sensor_Measurement_Object_1/2  "Object_ID[]"
  Object_Type[]/1(Out1) -> Custom_Sensor_Measurement_Object_1/3  "Object_Type[]"
  Bus Selector2/3 -> CustomSensor_Data_Valid[0|1]/1(In1)  "<CustomSensor_Data_Valid[0|1]>"
  CustomSensor_Data_Valid[0|1]/1(Out1) -> Custom_Sensor_Info/3  "CustomSensor_Data_Valid[0|1]"
  Bus Selector3/1 -> Bus Selector4/1  "<Object1>"
  Bus Selector4/7 -> CustomValues[]/1(In1)  "<CustomValues[]>"
  CustomValues[]/1(Out1) -> Custom_Sensor_Measurement_Object_1/7  "CustomValues[]"
  Angle_Ver_Rel[deg]1/1(Out1) -> Custom_Sensor_Measurement_Object_2/6  "Angle_Ver_Rel[deg]"
  Angle_Hor_Rel[deg]1/1(Out1) -> Custom_Sensor_Measurement_Object_2/5  "Angle_Hor_Rel[deg]"
  Distance[m]1/1(Out1) -> Custom_Sensor_Measurement_Object_2/4  "Distance[m]"
  Object_Valid[0|1]1/1(Out1) -> Custom_Sensor_Measurement_Object_2/1  "Object_Valid[0|1]"
  Bus Selector6/6 -> Angle_Ver_Rel[deg]1/1(In1)  "<Angle_Ver_Rel[deg]>"
  Bus Selector6/5 -> Angle_Hor_Rel[deg]1/1(In1)  "<Angle_Hor_Rel[deg]>"
  Bus Selector6/4 -> Distance[m]1/1(In1)  "<Distance[m]>"
  Bus Selector6/3 -> Object_Type[]1/1(In1)  "<Object_Type[]>"
  Bus Selector6/2 -> Object_ID[]1/1(In1)  "<Object_ID[]>"
  Bus Selector6/1 -> Object_Valid[0|1]1/1(In1)  "<Object_Valid[0|1]>"
  Object_ID[]1/1(Out1) -> Custom_Sensor_Measurement_Object_2/2  "Object_ID[]"
  Object_Type[]1/1(Out1) -> Custom_Sensor_Measurement_Object_2/3  "Object_Type[]"
  Bus Selector5/1 -> Bus Selector6/1  "<Object1>"
  Bus Selector6/7 -> CustomValues[]1/1(In1)  "<CustomValues[]>"
  CustomValues[]1/1(Out1) -> Custom_Sensor_Measurement_Object_2/7  "CustomValues[]"
